simulink model "Problem_2"  (R2020a)
settings: Solver=VariableStepAuto  StartTime=0.0  StopTime=10.0  RelTol=1e-3
undefined symbols (not defined in the file): b, k, k2
settings Model: Creator=Saqlain  LastModifiedBy=Saqlain

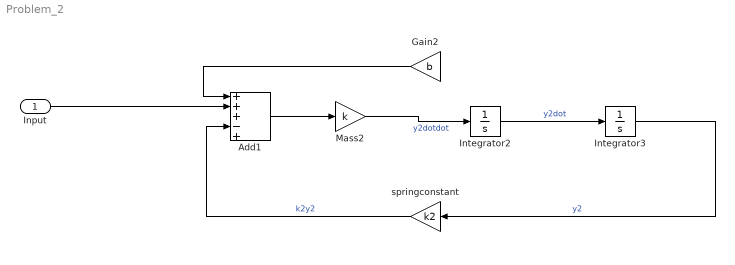
== system Problem_2 ==
  Input : Inport
  Add1 : Sum  Inputs=+++-+
  Gain2 : Gain  Gain=b
  Integrator2 : Integrator
  Integrator3 : Integrator
  Mass2 : Gain  Gain=k
  springconstant : Gain  Gain=k2
  wires:
  springconstant/1 -> Add1/4  "k2y2"
  Input/1 -> Add1/2
  Mass2/1 -> Integrator2/1  "y2dotdot"
  Gain2/1 -> Add1/1
  Integrator3/1 -> springconstant/1  "y2"
  Add1/1 -> Mass2/1
  Integrator2/1 -> Integrator3/1  "y2dot"
